simulink model "aero_control_dynamics_model"  (R2021a)
settings: Solver=FixedStepAuto  StartTime=0.0  StopTime=10.0  FixedStep=T_sample_control  RelTol=1e-3
InitFcn:
  | aero_control_dynamics_config
values from neighbouring files (symbols this model uses):
  pitch_force = readtable('pitch_force.csv')    [aero_control_dynamics_config.m]
  pitch_moment = readtable('pitch_moment.csv')    [aero_control_dynamics_config.m]
  roll_force = readtable('roll_force.csv')    [aero_control_dynamics_config.m]
  roll_moment = readtable('roll_moment.csv')    [aero_control_dynamics_config.m]
  yaw_force = readtable('yaw_force.csv')    [aero_control_dynamics_config.m]
  yaw_moment = readtable('yaw_moment.csv')    [aero_control_dynamics_config.m]
undefined symbols (not defined in the file or in its folder): gf2N, K_w_F, K_w_M, Nmm2Nm
settings Model: DataDictionary=pid.sldd  Creator=Nabil  LastModifiedBy=jadg1

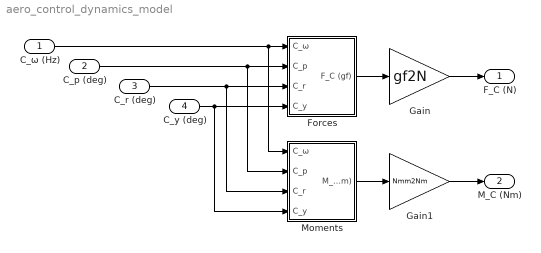
== system aero_control_dynamics_model ==
  C_ω (Hz) : Inport
  C_p (deg) : Inport  Port=2
  C_r (deg) : Inport  Port=3
  C_y (deg) : Inport  Port=4
  Forces : Subsystem
  Gain : Gain  Gain=gf2N
  Gain1 : Gain  Gain=Nmm2Nm
  Moments : Subsystem
  F_C (N) : Outport
  M_C (Nm) : Outport  Port=2
  wires:
  Forces/1(F_C (gf)) -> Gain/1
  Gain1/1 -> M_C (Nm)/1
  C_y (deg)/1 -> Moments/4(C_y), Forces/4(C_y)
  Moments/1(M_C (Nmm)) -> Gain1/1
  Gain/1 -> F_C (N)/1
  C_p (deg)/1 -> Moments/2(C_p), Forces/2(C_p)
  C_r (deg)/1 -> Moments/3(C_r), Forces/3(C_r)
  C_ω (Hz)/1 -> Forces/1(C_ω), Moments/1(C_ω)

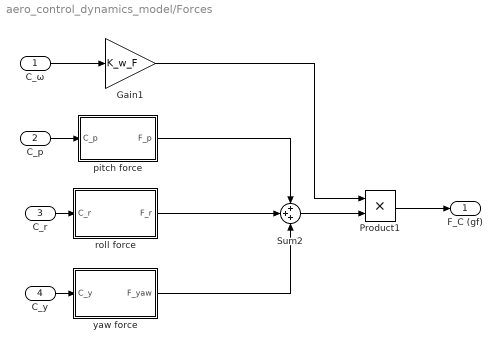
== system aero_control_dynamics_model/Forces ==
  C_ω : Inport
  C_p : Inport  Port=2
  C_r : Inport  Port=3
  C_y : Inport  Port=4
  Gain1 : Gain  Gain=K_w_F
  Product1 : Product
  Sum2 : Sum  Inputs=+++
  pitch force : Subsystem
  roll force : Subsystem
  yaw force : Subsystem
  F_C (gf) : Outport
  wires:
  roll force/1(F_r) -> Sum2/2
  C_p/1 -> pitch force/1(C_p)
  pitch force/1(F_p) -> Sum2/1
  Sum2/1 -> Product1/2
  yaw force/1(F_yaw) -> Sum2/3
  Product1/1 -> F_C (gf)/1
  C_y/1 -> yaw force/1(C_y)
  Gain1/1 -> Product1/1
  C_r/1 -> roll force/1(C_r)
  C_ω/1 -> Gain1/1

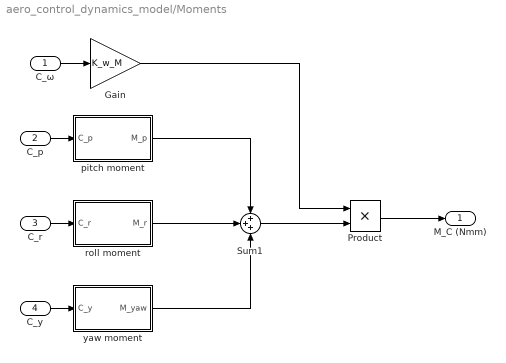
== system aero_control_dynamics_model/Moments ==
  C_ω : Inport
  C_p : Inport  Port=2
  C_r : Inport  Port=3
  C_y : Inport  Port=4
  Gain : Gain  Gain=K_w_M
  Product : Product
  Sum1 : Sum  Inputs=+++
  pitch moment : Subsystem
  roll moment : Subsystem
  yaw moment : Subsystem
  M_C (Nmm) : Outport
  wires:
  Sum1/1 -> Product/2
  yaw moment/1(M_yaw) -> Sum1/3
  Gain/1 -> Product/1
  roll moment/1(M_r) -> Sum1/2
  Product/1 -> M_C (Nmm)/1
  C_y/1 -> yaw moment/1(C_y)
  pitch moment/1(M_p) -> Sum1/1
  C_p/1 -> pitch moment/1(C_p)
  C_r/1 -> roll moment/1(C_r)
  C_ω/1 -> Gain/1

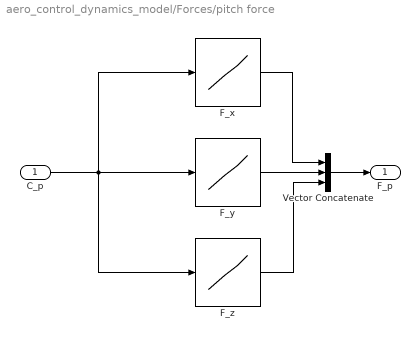
== system aero_control_dynamics_model/Forces/pitch force ==
  C_p : Inport
  F_x : Lookup_n-D  NumberOfTableDimensions=1  BreakpointsForDimension1="pitch_force.(\"command\")"  BreakpointsForDimension2="pitch_force.(\"command\")"  BreakpointsForDimension3="pitch_force.(\"command\")"  BreakpointsForDimension4="pitch_force.(\"command\")"  BreakpointsForDimension1FirstPoint=-15  BreakpointsForDimension2FirstPoint=15  BreakpointsForDimension1Spacing=7.5  Table="pitch_force.(\"F_x\")"  DiagnosticForOutOfRangeInput=Error  InternalRulePriority=Speed  RndMeth=Simplest  InputSameDT=on
  F_y : Lookup_n-D  NumberOfTableDimensions=1  BreakpointsForDimension1="pitch_force.(\"command\")"  BreakpointsForDimension2="pitch_force.(\"command\")"  BreakpointsForDimension3="pitch_force.(\"command\")"  BreakpointsForDimension4="pitch_force.(\"command\")"  BreakpointsForDimension1FirstPoint=-15  BreakpointsForDimension2FirstPoint=15  BreakpointsForDimension1Spacing=7.5  Table="pitch_force.(\"F_y\")"  DiagnosticForOutOfRangeInput=Error  InternalRulePriority=Speed  RndMeth=Simplest  InputSameDT=on
  F_z : Lookup_n-D  NumberOfTableDimensions=1  BreakpointsForDimension1="pitch_force.(\"command\")"  BreakpointsForDimension2="pitch_force.(\"command\")"  BreakpointsForDimension3="pitch_force.(\"command\")"  BreakpointsForDimension4="pitch_force.(\"command\")"  BreakpointsForDimension1FirstPoint=-15  BreakpointsForDimension2FirstPoint=15  BreakpointsForDimension1Spacing=7.5  Table="pitch_force.(\"F_z\")"  DiagnosticForOutOfRangeInput=Error  InternalRulePriority=Speed  RndMeth=Simplest  InputSameDT=on
  Vector Concatenate : Concatenate  NumInputs=3
  F_p : Outport
  wires:
  F_z/1 -> Vector Concatenate/3
  C_p/1 -> F_z/1, F_x/1, F_y/1
  F_x/1 -> Vector Concatenate/1
  Vector Concatenate/1 -> F_p/1
  F_y/1 -> Vector Concatenate/2

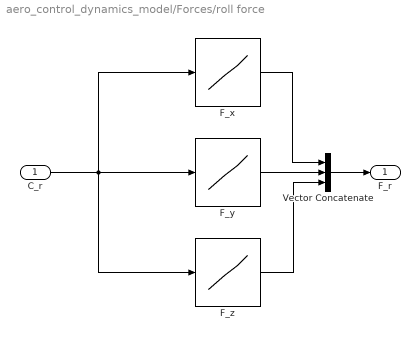
== system aero_control_dynamics_model/Forces/roll force ==
  C_r : Inport
  F_x : Lookup_n-D  NumberOfTableDimensions=1  BreakpointsForDimension1="roll_force.(\"command\")"  BreakpointsForDimension2="pitch_force.(\"command\")"  BreakpointsForDimension3="pitch_force.(\"command\")"  BreakpointsForDimension4="pitch_force.(\"command\")"  BreakpointsForDimension1FirstPoint=-15  BreakpointsForDimension2FirstPoint=15  BreakpointsForDimension1Spacing=7.5  Table="roll_force.(\"F_x\")"  DiagnosticForOutOfRangeInput=Error  InternalRulePriority=Speed  RndMeth=Simplest  InputSameDT=on
  F_y : Lookup_n-D  NumberOfTableDimensions=1  BreakpointsForDimension1="roll_force.(\"command\")"  BreakpointsForDimension2="pitch_force.(\"command\")"  BreakpointsForDimension3="pitch_force.(\"command\")"  BreakpointsForDimension4="pitch_force.(\"command\")"  BreakpointsForDimension1FirstPoint=-15  BreakpointsForDimension2FirstPoint=15  BreakpointsForDimension1Spacing=7.5  Table="roll_force.(\"F_y\")"  DiagnosticForOutOfRangeInput=Error  InternalRulePriority=Speed  RndMeth=Simplest  InputSameDT=on
  F_z : Lookup_n-D  NumberOfTableDimensions=1  BreakpointsForDimension1="roll_force.(\"command\")"  BreakpointsForDimension2="pitch_force.(\"command\")"  BreakpointsForDimension3="pitch_force.(\"command\")"  BreakpointsForDimension4="pitch_force.(\"command\")"  BreakpointsForDimension1FirstPoint=-15  BreakpointsForDimension2FirstPoint=15  BreakpointsForDimension1Spacing=7.5  Table="roll_force.(\"F_z\")"  DiagnosticForOutOfRangeInput=Error  InternalRulePriority=Speed  RndMeth=Simplest  InputSameDT=on
  Vector Concatenate : Concatenate  NumInputs=3
  F_r : Outport
  wires:
  F_z/1 -> Vector Concatenate/3
  C_r/1 -> F_z/1, F_x/1, F_y/1
  F_x/1 -> Vector Concatenate/1
  Vector Concatenate/1 -> F_r/1
  F_y/1 -> Vector Concatenate/2

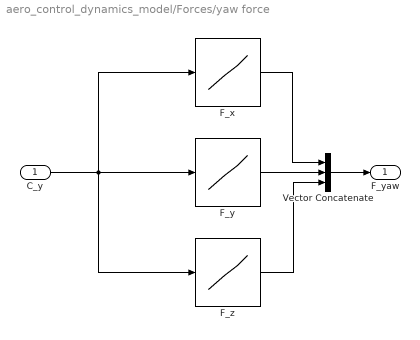
== system aero_control_dynamics_model/Forces/yaw force ==
  C_y : Inport
  F_x : Lookup_n-D  NumberOfTableDimensions=1  BreakpointsForDimension1="yaw_force.(\"command\")"  BreakpointsForDimension2="pitch_force.(\"command\")"  BreakpointsForDimension3="pitch_force.(\"command\")"  BreakpointsForDimension4="pitch_force.(\"command\")"  BreakpointsForDimension1FirstPoint=-15  BreakpointsForDimension2FirstPoint=15  BreakpointsForDimension1Spacing=7.5  Table="yaw_force.(\"F_x\")"  DiagnosticForOutOfRangeInput=Error  InternalRulePriority=Speed  RndMeth=Simplest  InputSameDT=on
  F_y : Lookup_n-D  NumberOfTableDimensions=1  BreakpointsForDimension1="yaw_force.(\"command\")"  BreakpointsForDimension2="pitch_force.(\"command\")"  BreakpointsForDimension3="pitch_force.(\"command\")"  BreakpointsForDimension4="pitch_force.(\"command\")"  BreakpointsForDimension1FirstPoint=-15  BreakpointsForDimension2FirstPoint=15  BreakpointsForDimension1Spacing=7.5  Table="yaw_force.(\"F_y\")"  DiagnosticForOutOfRangeInput=Error  InternalRulePriority=Speed  RndMeth=Simplest  InputSameDT=on
  F_z : Lookup_n-D  NumberOfTableDimensions=1  BreakpointsForDimension1="yaw_force.(\"command\")"  BreakpointsForDimension2="pitch_force.(\"command\")"  BreakpointsForDimension3="pitch_force.(\"command\")"  BreakpointsForDimension4="pitch_force.(\"command\")"  BreakpointsForDimension1FirstPoint=-15  BreakpointsForDimension2FirstPoint=15  BreakpointsForDimension1Spacing=7.5  Table="yaw_force.(\"F_z\")"  DiagnosticForOutOfRangeInput=Error  InternalRulePriority=Speed  RndMeth=Simplest  InputSameDT=on
  Vector Concatenate : Concatenate  NumInputs=3
  F_yaw : Outport
  wires:
  F_z/1 -> Vector Concatenate/3
  C_y/1 -> F_z/1, F_x/1, F_y/1
  F_x/1 -> Vector Concatenate/1
  Vector Concatenate/1 -> F_yaw/1
  F_y/1 -> Vector Concatenate/2

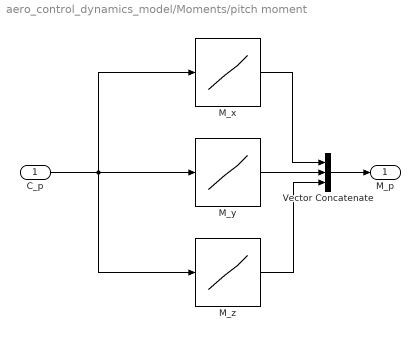
== system aero_control_dynamics_model/Moments/pitch moment ==
  C_p : Inport
  M_x : Lookup_n-D  NumberOfTableDimensions=1  BreakpointsForDimension1="pitch_moment.(\"command\")"  BreakpointsForDimension2="pitch_force.(\"command\")"  BreakpointsForDimension3="pitch_force.(\"command\")"  BreakpointsForDimension4="pitch_force.(\"command\")"  BreakpointsForDimension1FirstPoint=-15  BreakpointsForDimension2FirstPoint=15  BreakpointsForDimension1Spacing=7.5  Table="pitch_moment.(\"M_x\")"  DiagnosticForOutOfRangeInput=Error  InternalRulePriority=Speed  RndMeth=Simplest  InputSameDT=on
  M_y : Lookup_n-D  NumberOfTableDimensions=1  BreakpointsForDimension1="pitch_moment.(\"command\")"  BreakpointsForDimension2="pitch_force.(\"command\")"  BreakpointsForDimension3="pitch_force.(\"command\")"  BreakpointsForDimension4="pitch_force.(\"command\")"  BreakpointsForDimension1FirstPoint=-15  BreakpointsForDimension2FirstPoint=15  BreakpointsForDimension1Spacing=7.5  Table="pitch_moment.(\"M_y\")"  DiagnosticForOutOfRangeInput=Error  InternalRulePriority=Speed  RndMeth=Simplest  InputSameDT=on
  M_z : Lookup_n-D  NumberOfTableDimensions=1  BreakpointsForDimension1="pitch_moment.(\"command\")"  BreakpointsForDimension2="pitch_force.(\"command\")"  BreakpointsForDimension3="pitch_force.(\"command\")"  BreakpointsForDimension4="pitch_force.(\"command\")"  BreakpointsForDimension1FirstPoint=-15  BreakpointsForDimension2FirstPoint=15  BreakpointsForDimension1Spacing=7.5  Table="pitch_moment.(\"M_z\")"  DiagnosticForOutOfRangeInput=Error  InternalRulePriority=Speed  RndMeth=Simplest  InputSameDT=on
  Vector Concatenate : Concatenate  NumInputs=3
  M_p : Outport
  wires:
  M_z/1 -> Vector Concatenate/3
  C_p/1 -> M_z/1, M_x/1, M_y/1
  M_x/1 -> Vector Concatenate/1
  Vector Concatenate/1 -> M_p/1
  M_y/1 -> Vector Concatenate/2

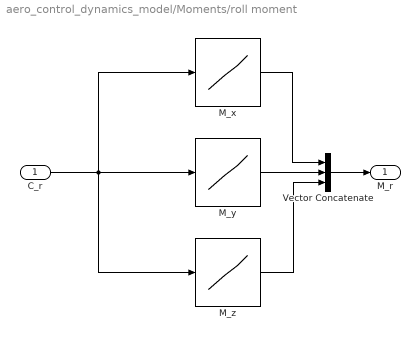
== system aero_control_dynamics_model/Moments/roll moment ==
  C_r : Inport
  M_x : Lookup_n-D  NumberOfTableDimensions=1  BreakpointsForDimension1="roll_moment.(\"command\")"  BreakpointsForDimension2="pitch_force.(\"command\")"  BreakpointsForDimension3="pitch_force.(\"command\")"  BreakpointsForDimension4="pitch_force.(\"command\")"  BreakpointsForDimension1FirstPoint=-15  BreakpointsForDimension2FirstPoint=15  BreakpointsForDimension1Spacing=7.5  Table="roll_moment.(\"M_x\")"  DiagnosticForOutOfRangeInput=Error  InternalRulePriority=Speed  RndMeth=Simplest  InputSameDT=on
  M_y : Lookup_n-D  NumberOfTableDimensions=1  BreakpointsForDimension1="roll_moment.(\"command\")"  BreakpointsForDimension2="pitch_force.(\"command\")"  BreakpointsForDimension3="pitch_force.(\"command\")"  BreakpointsForDimension4="pitch_force.(\"command\")"  BreakpointsForDimension1FirstPoint=-15  BreakpointsForDimension2FirstPoint=15  BreakpointsForDimension1Spacing=7.5  Table="roll_moment.(\"M_y\")"  DiagnosticForOutOfRangeInput=Error  InternalRulePriority=Speed  RndMeth=Simplest  InputSameDT=on
  M_z : Lookup_n-D  NumberOfTableDimensions=1  BreakpointsForDimension1="roll_moment.(\"command\")"  BreakpointsForDimension2="pitch_force.(\"command\")"  BreakpointsForDimension3="pitch_force.(\"command\")"  BreakpointsForDimension4="pitch_force.(\"command\")"  BreakpointsForDimension1FirstPoint=-15  BreakpointsForDimension2FirstPoint=15  BreakpointsForDimension1Spacing=7.5  Table="roll_moment.(\"M_z\")"  DiagnosticForOutOfRangeInput=Error  InternalRulePriority=Speed  RndMeth=Simplest  InputSameDT=on
  Vector Concatenate : Concatenate  NumInputs=3
  M_r : Outport
  wires:
  M_z/1 -> Vector Concatenate/3
  C_r/1 -> M_z/1, M_x/1, M_y/1
  M_x/1 -> Vector Concatenate/1
  Vector Concatenate/1 -> M_r/1
  M_y/1 -> Vector Concatenate/2

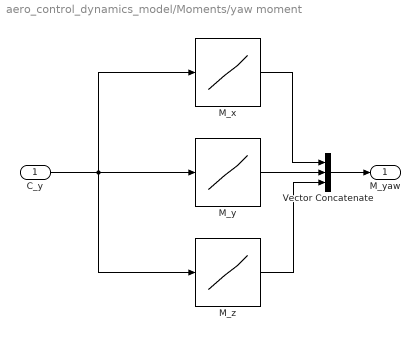
== system aero_control_dynamics_model/Moments/yaw moment ==
  C_y : Inport
  M_x : Lookup_n-D  NumberOfTableDimensions=1  BreakpointsForDimension1="yaw_moment.(\"command\")"  BreakpointsForDimension2="pitch_force.(\"command\")"  BreakpointsForDimension3="pitch_force.(\"command\")"  BreakpointsForDimension4="pitch_force.(\"command\")"  BreakpointsForDimension1FirstPoint=-15  BreakpointsForDimension2FirstPoint=15  BreakpointsForDimension1Spacing=7.5  Table="yaw_moment.(\"M_x\")"  DiagnosticForOutOfRangeInput=Error  InternalRulePriority=Speed  RndMeth=Simplest  InputSameDT=on
  M_y : Lookup_n-D  NumberOfTableDimensions=1  BreakpointsForDimension1="yaw_moment.(\"command\")"  BreakpointsForDimension2="pitch_force.(\"command\")"  BreakpointsForDimension3="pitch_force.(\"command\")"  BreakpointsForDimension4="pitch_force.(\"command\")"  BreakpointsForDimension1FirstPoint=-15  BreakpointsForDimension2FirstPoint=15  BreakpointsForDimension1Spacing=7.5  Table="yaw_moment.(\"M_y\")"  DiagnosticForOutOfRangeInput=Error  InternalRulePriority=Speed  RndMeth=Simplest  InputSameDT=on
  M_z : Lookup_n-D  NumberOfTableDimensions=1  BreakpointsForDimension1="yaw_moment.(\"command\")"  BreakpointsForDimension2="pitch_force.(\"command\")"  BreakpointsForDimension3="pitch_force.(\"command\")"  BreakpointsForDimension4="pitch_force.(\"command\")"  BreakpointsForDimension1FirstPoint=-15  BreakpointsForDimension2FirstPoint=15  BreakpointsForDimension1Spacing=7.5  Table="yaw_moment.(\"M_z\")"  DiagnosticForOutOfRangeInput=Error  InternalRulePriority=Speed  RndMeth=Simplest  InputSameDT=on
  Vector Concatenate : Concatenate  NumInputs=3
  M_yaw : Outport
  wires:
  M_z/1 -> Vector Concatenate/3
  C_y/1 -> M_z/1, M_x/1, M_y/1
  M_x/1 -> Vector Concatenate/1
  Vector Concatenate/1 -> M_yaw/1
  M_y/1 -> Vector Concatenate/2
